simulink model "model"  (R2024a)
settings: Solver=VariableStepAuto  StartTime=0.0  StopTime=simulation_time  RelTol=1e-3
values from neighbouring files (symbols this model uses):
  dq_0 = zeros(n, 1)    [example.m]
  path = @(t) circle_center + u_circle_plane*radius*cos((t/T) * (2*pi)) + v_circle_plane*radius*sin((t/T) * (2*pi))    [example.m]
  path_ddot = @(t) -u_circle_plane*radius*(2*pi/T)*(2*pi/T)*cos((t/T) * (2*pi)) - v_circle_plane*radius*(2*pi/T)*(2*pi/T)*sin((t/T) * (2*pi))    [example.m]
  path_dot = @(t) -u_circle_plane*radius*(2*pi/T)*sin((t/T) * (2*pi)) + v_circle_plane*radius*(2*pi/T)*cos((t/T) * (2*pi))    [example.m]
  q_0 = randn(n, 1)    [example.m]
libraries: robotmaniplib x2
settings Model: Creator=pietro  LastModifiedBy=salvatore

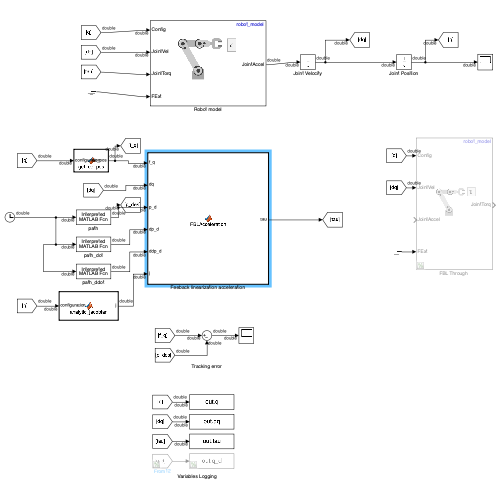
[thumbnail: Simulink's stored preview of the top-level diagram]
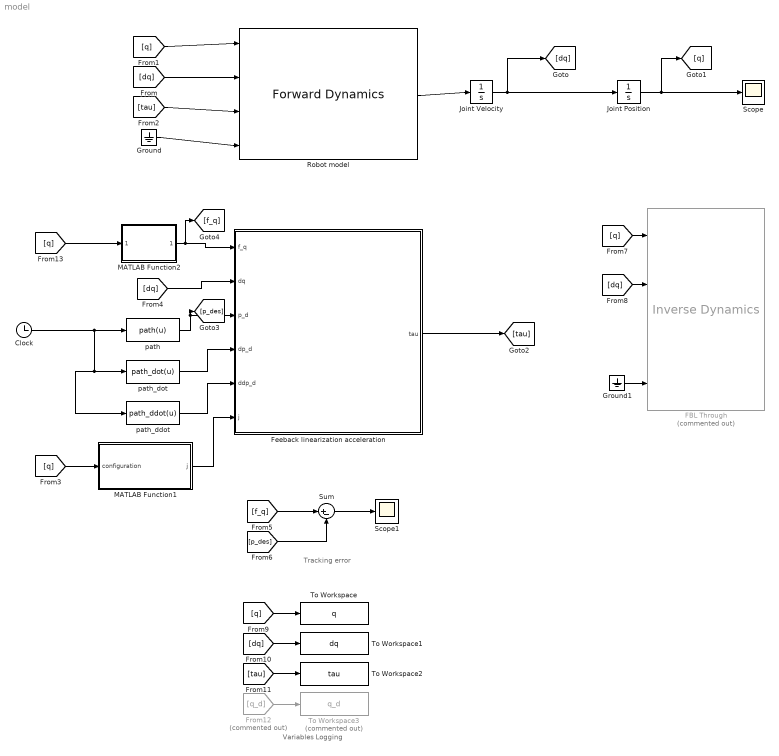
== system model ==
  note: Variables Logging
  note: Tracking error
  Clock : Clock
  "FBL Through " : robotmaniplib/Inverse Dynamics  Commented=on  RigidBodyTree=robot_model  SimulateUsing=Code generation
  Feeback linearization acceleration : MATLAB Function  TreatAsAtomicUnit=on
  From12 : From  Commented=on  GotoTag=q_d
  Ground : Ground
  Ground1 : Ground
  Joint Position : Integrator  InitialCondition=q_0
  Joint Velocity : Integrator  InitialCondition=dq_0
  MATLAB Function1 : MATLAB Function  TreatAsAtomicUnit=on
  MATLAB Function2 : MATLAB Function  TreatAsAtomicUnit=on
  Robot model : robotmaniplib/Forward Dynamics  RigidBodyTree=robot_model  SimulateUsing=Code generation
  Scope : Scope
  Scope1 : Scope
  Sum : Sum  Inputs=|+-
  To Workspace : ToWorkspace  VariableName=q  SaveFormat=Timeseries  SampleTime=-1
  To Workspace1 : ToWorkspace  VariableName=dq  SaveFormat=Timeseries  SampleTime=-1
  To Workspace2 : ToWorkspace  VariableName=tau  SaveFormat=Timeseries  SampleTime=-1
  To Workspace3 : ToWorkspace  Commented=on  VariableName=q_d  SaveFormat=Timeseries  SampleTime=-1
  path : MATLABFcn  MATLABFcn=path(u)
  path_ddot : MATLABFcn  MATLABFcn=path_ddot(u)
  path_dot : MATLABFcn  MATLABFcn=path_dot(u)
  wires:
  Robot model/1 -> Joint Velocity/1
  Joint Velocity/1 -> [dq], Joint Position/1
  [dq] -> Robot model/2
  Joint Position/1 -> Scope/1, [q]
  [q] -> Robot model/1
  [tau] -> Robot model/3
  Ground/1 -> Robot model/4
  MATLAB Function2/1(ee_pos) -> [f_q], Feeback linearization acceleration/1(f_q)
  [dq] -> Feeback linearization acceleration/2(dq)
  path/1 -> [p_des], Feeback linearization acceleration/3(p_d)
  Clock/1 -> path_ddot/1, path_dot/1, path/1
  path_dot/1 -> Feeback linearization acceleration/4(dp_d)
  path_ddot/1 -> Feeback linearization acceleration/5(ddp_d)
  [f_q] -> Sum/1
  [p_des] -> Sum/2
  Sum/1 -> Scope1/1
  [q] -> "FBL Through "/1
  [dq] -> "FBL Through "/2
  Ground1/1 -> "FBL Through "/4
  [q] -> To Workspace/1
  [dq] -> To Workspace1/1
  [tau] -> To Workspace2/1
  From12/1 -> To Workspace3/1
  [q] -> MATLAB Function2/1(configuration)
  MATLAB Function1/1(j) -> Feeback linearization acceleration/6(j)
  [q] -> MATLAB Function1/1(configuration)
  Feeback linearization acceleration/1(tau) -> [tau]

== matlab function model/Feeback linearization acceleration ==
  data: f_q input; tau output; dq input; p_d input; dp_d input; ddp_d input; j input
function tau = FBLAcceleration(f_q, dq, p_d, dp_d, ddp_d, j)

% Control gains
K_P = 100;
K_D = 10;

% Acceleration command of the FBL controller
% a   = ddq_d + K_P*(q_d - q) + K_D*(dq_d - dq);
disp(size(j));
disp(size(dq));
disp(size(p_d));

tau = j' * K_P * (p_d - f_q) + K_D * (pinv(j)*dp_d - dq);

end

== matlab function model/MATLAB Function1 ==
  data: configuration input; j output
function j = analytic_jacobian(configuration)
%ANALYTIC_JACOBIAN1
%    J = ANALYTIC_JACOBIAN1(Q1,Q2,Q3,Q4)

%    This function was generated by the Symbolic Math Toolbox version 24.1.
%    02-Jul-2024 11:08:16

q1 = configuration(1);
q2 = configuration(2);
q3 = configuration(3);
q4 = configuration(4);

t2 = cos(q1);
t3 = cos(q2);
t4 = cos(q3);
t5 = cos(q4);
t6 = sin(q1);
t7 = sin(q2);
t8 = sin(q3);
t9 = sin(q4);
t10 = t2.*t8;
t11 = t6.*t8;
t12 = t2.*t3.*t4;
t13 = t3.*t4.*t6;
t14 = -t12;
t15 = t10+t13;
t16 = t11+t14;
mt1 = [t6.*t7.*(2.0./5.0)-t9.*t15.*(3.9e+1./1.0e+2)+t5.*t6.*t7.*(3.9e+1./1.0e+2),t2.*t7.*(-2.0./5.0)-t9.*t16.*(3.9e+1./1.0e+2)-t2.*t5.*t7.*(3.9e+1./1.0e+2),0.0,t2.*t3.*(-2.0./5.0)-t2.*t3.*t5.*(3.9e+1./1.0e+2)-t2.*t4.*t7.*t9.*(3.9e+1./1.0e+2),t3.*t6.*(-2.0./5.0)-t3.*t5.*t6.*(3.9e+1./1.0e+2)-t4.*t6.*t7.*t9.*(3.9e+1./1.0e+2),t7.*(-2.0./5.0)-t5.*t7.*(3.9e+1./1.0e+2)+t3.*t4.*t9.*(3.9e+1./1.0e+2),t9.*(t4.*t6+t3.*t10).*(-3.9e+1./1.0e+2),t9.*(t2.*t4-t3.*t11).*(3.9e+1./1.0e+2),t7.*t8.*t9.*(-3.9e+1./1.0e+2)];
mt2 = [t5.*t16.*(-3.9e+1./1.0e+2)+t2.*t7.*t9.*(3.9e+1./1.0e+2),t5.*t15.*(3.9e+1./1.0e+2)+t6.*t7.*t9.*(3.9e+1./1.0e+2),t3.*t9.*(-3.9e+1./1.0e+2)+t4.*t5.*t7.*(3.9e+1./1.0e+2),0.0,0.0,0.0,0.0,0.0,0.0,0.0,0.0,0.0];
j = reshape([mt1,mt2],3,7);
end

== matlab function model/MATLAB Function2 ==
  data: configuration input; ee_pos output
% function A0e = get_ee_pos(configuration)
function ee_pos = get_ee_pos(configuration)
%F_Q1
%    OUT1 = F_Q1(Q1,Q2,Q3,Q4)

%    This function was generated by the Symbolic Math Toolbox version 24.1.
%    02-Jul-2024 11:07:49
q1 = configuration(1);
q2 = configuration(2);
q3 = configuration(3);
q4 = configuration(4);

t2 = cos(q1);
t3 = cos(q2);
t4 = cos(q3);
t5 = cos(q4);
t6 = sin(q1);
t7 = sin(q2);
t8 = sin(q3);
t9 = sin(q4);
ee_pos = [t9.*(t6.*t8-t2.*t3.*t4).*(-3.9e+1./1.0e+2)-t2.*t7.*(2.0./5.0)-t2.*t5.*t7.*(3.9e+1./1.0e+2);t9.*(t2.*t8+t3.*t4.*t6).*(3.9e+1./1.0e+2)-t6.*t7.*(2.0./5.0)-t5.*t6.*t7.*(3.9e+1./1.0e+2);t3.*(2.0./5.0)+t3.*t5.*(3.9e+1./1.0e+2)+t4.*t7.*t9.*(3.9e+1./1.0e+2)+3.1e+1./1.0e+2];
end
